simulink model "red_atraso"  (R2020b)
settings: Solver=VariableStepAuto  StartTime=0.0  StopTime=70  RelTol=1e-3
values from neighbouring files (symbols this model uses):
  den = conv([1 p1],[1 p2])    [adelanto_atraso_ej.m]
  Kc = 20    [adelanto_atraso_ej.m]    (also in adelanto_fase.m = K/a)
  p = 1/(T*a)    [adelanto_fase.m]
  z = 1/T    [adelanto_fase.m]
libraries: simulink x2
settings Model: Creator=Acer  LastModifiedBy=Acer

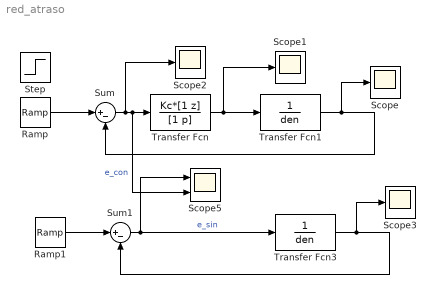
== system red_atraso ==
  Ramp : simulink/Sources/Ramp  slope=1  start=0  InitialOutput=0
  Ramp1 : simulink/Sources/Ramp  slope=1  start=0  InitialOutput=0
  Scope{,1..3} (4 alike) : Scope
  Scope5 : Scope  NumInputPorts=2
  Step : Step  Time=0  SampleTime=0
  Sum : Sum  Inputs=|+-
  Sum1 : Sum  Inputs=|+-
  Transfer Fcn : TransferFcn  Numerator=Kc*[1 z]  Denominator=[1 p]
  Transfer Fcn1 : TransferFcn  Numerator=1  Denominator=den
  Transfer Fcn3 : TransferFcn  Numerator=1  Denominator=den
  wires:
  Sum/1 -> Scope2/1, Scope5/2, Transfer Fcn/1  "e_con"
  Transfer Fcn/1 -> Scope1/1, Transfer Fcn1/1
  Transfer Fcn1/1 -> Scope/1, Sum/2
  Ramp/1 -> Sum/1
  Ramp1/1 -> Sum1/1
  Transfer Fcn3/1 -> Scope3/1, Sum1/2
  Sum1/1 -> Transfer Fcn3/1, Scope5/1  "e_sin"
